simulink model "Balancing Model"  (R2024a)
settings: Solver=VariableStepAuto  StartTime=0.0  StopTime=inf  RelTol=1e-3
settings Model: Creator=Ganna Ayman  LastModifiedBy=Ganna Ayman

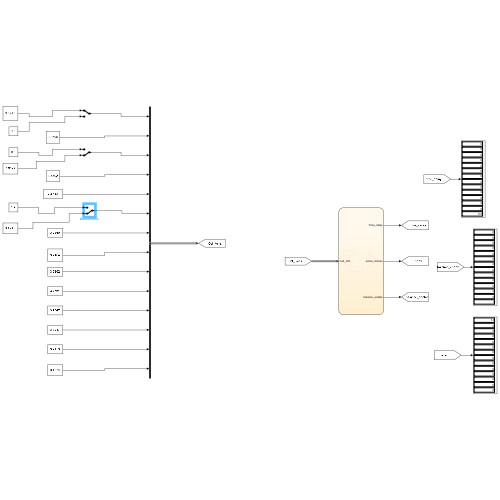
[thumbnail: Simulink's stored preview of the top-level diagram]
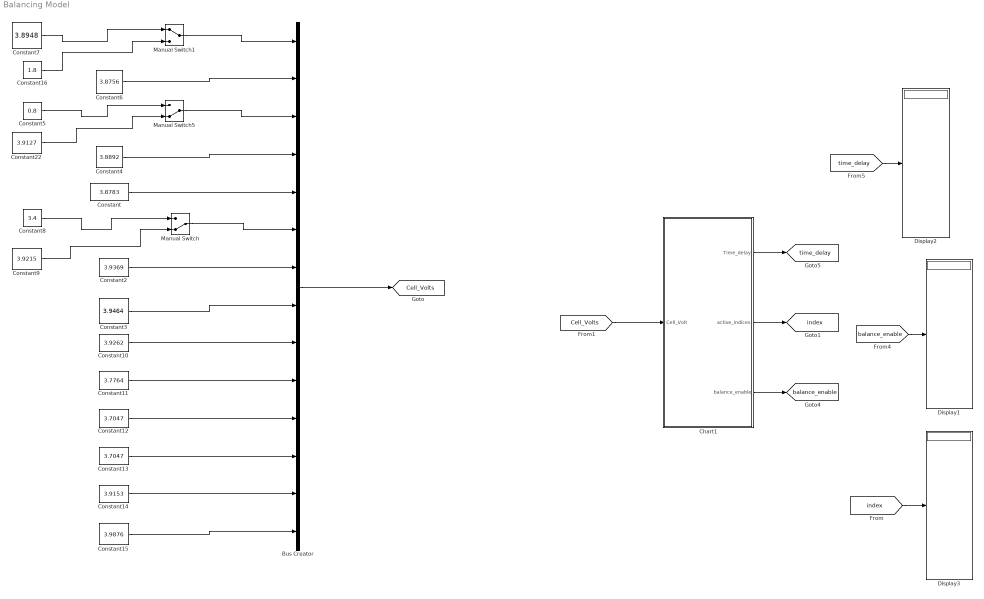
== system Balancing Model ==
  Bus Creator : BusCreator  Inputs=14
  Chart1 : Stateflow chart  TreatAsAtomicUnit=on
      settings: PortSchema="{\"entries\":[{\"content\":{\"sides\":[{\"content\":{\"connectorIds\":[\"In1\"]},\"type\":\"ConnectorPlacement.EquallySpacedRectSide\",\"uuid\":\"6f312cc7-79af-4024-8579-3732173f9295\"},{\"content\":{\"connectorIds\":[\"Out2\",\"Out3\",\"Out1\"],\"side\":\"RIGHT\"},\"type\":\"ConnectorPlacement.EquallySpacedRectSide\",\"uuid\":\"3dc9c74e-fd1a-461c-96fc-bb153941e7b5\"},{\"content\":{\"side\":\"TOP\"},\"type\":\"ConnectorPlacement.EquallySpacedRectSide\",\"uuid\":\"e4504d25-18f4-45f4-b711-d682a6c51dcf\"}]},\"type\":\"ConnectorPlacement.EquallySpacedConnector\",\"uuid\":\"9caf59e1-89f7-43be-b634-7a97cd583662\"}],\"packageUris\":[\"http://schema.mathworks.com/mf0/Connector/R2020b\"],\"version\":\"1.0\"}"
  Constant : Constant  Value=3.8783
  Constant10 : Constant  Value=3.9262
  Constant11 : Constant  Value=3.7764
  Constant12 : Constant  Value=3.7047
  Constant13 : Constant  Value=3.7047
  Constant14 : Constant  Value=3.9153
  Constant15 : Constant  Value=3.9876
  Constant16 : Constant  Value=1.8
  Constant2 : Constant  Value=3.9369
  Constant22 : Constant  Value=3.9127
  Constant3 : Constant  Value=3.9464
  Constant4 : Constant  Value=3.8892
  Constant5 : Constant  Value=0.8
  Constant6 : Constant  Value=3.8756
  Constant7 : Constant  Value=3.8948
  Constant8 : Constant  Value=3.4
  Constant9 : Constant  Value=3.9215
  Display1 : Display
  Display2 : Display
  Display3 : Display
  Manual Switch : ManualSwitch  CurrentSetting=0
  Manual Switch1 : ManualSwitch
  Manual Switch5 : ManualSwitch  CurrentSetting=0
  tag scope: Cell_Volts=global, balance_enable=global, index=global, time_delay=global
  wires:
  Constant8/1 -> Manual Switch/1
  [balance_enable] -> Display1/1
  Constant10/1 -> Bus Creator/9
  Constant5/1 -> Manual Switch5/1
  [time_delay] -> Display2/1
  Constant4/1 -> Bus Creator/4
  Chart1/1(balance_enable) -> [balance_enable]
  Constant2/1 -> Bus Creator/7
  Manual Switch/1 -> Bus Creator/6
  Constant16/1 -> Manual Switch1/2
  Constant/1 -> Bus Creator/5
  Constant12/1 -> Bus Creator/11
  Bus Creator/1 -> [Cell_Volts]
  Constant3/1 -> Bus Creator/8
  Constant6/1 -> Bus Creator/2
  Constant11/1 -> Bus Creator/10
  Constant13/1 -> Bus Creator/12
  Constant7/1 -> Manual Switch1/1
  Constant15/1 -> Bus Creator/14
  Constant9/1 -> Manual Switch/2
  Constant14/1 -> Bus Creator/13
  Constant22/1 -> Manual Switch5/2
  Manual Switch5/1 -> Bus Creator/3
  Manual Switch1/1 -> Bus Creator/1
  Chart1/2(Time_delay) -> [time_delay]
  [index] -> Display3/1
  Chart1/3(active_indices) -> [index]
  [Cell_Volts] -> Chart1/1(Cell_Volt)

== stateflow chart Balancing Model/Chart1 ==
  state Discharge_Time_interval
    H= 1;
    Time_delay = zeros(1, 14);  % Initialize array
    during:
    for H = 1:14
    if balance_enable(H) == 1
    Time_delay(H) = 0.5; % 0.5min
    else
    Time_delay(H) = 0;      % 0 if disabled
    end
    end
    exit:
    H=1;
  state initialization
    entry:
    balance_enable=zeros(1,14);
    n=1;
    i=1;
    G=1;
    H=1;
  state Get_balance_reference
    entry:
    i=1
    cell_reference=10;
    during :
    for i = 1:14
    if (Cell_Volt(i) < cell_reference) && (Cell_Volt(i)>1.5)
    cell_reference = Cell_Volt(i);
    end
    end;
    exit:
    i=1;
  state Index_number
    entry:
    active_indices = zeros(1,14);  % Initialize output
    idx = 1;                     % Counter for active indices
    during:
    for G = 1:14
    if balance_enable(G) == 1
    active_indices(idx) = G;  % Store cell
    idx = idx + 1;
    end
    end
    exit:
    G=1;
  state Data_Check
    i = 1;
    % Main loop
    for i = 1:14
    if (Cell_Volt(i) > cell_reference) && (Cell_Volt(i) > 1.6) &&(Cell_Volt(i) - cell_reference > 0.25)
    balance_enable(i) = 1;
    else
    balance_enable(i) = 0; %had5ol feha 3and as8ar wa7da + lo el difference kan akber mn 0.25
    end
    end
    exit :
    i=1;
  state Error_Check
    entry:
    abdullah = 0;  % Initialize output (0 by default)
    during:
    for G = 1:14
    % Calculate absolute difference
    diff = abs(Cell_Volt(G) - cell_reference);
    % Check condition
    if diff > 0.5
    abdullah = 1;  % Set flag
    end
    end
    end
    exit:
    G=1;
  (default) -> initialization
  Discharge_Time_interval -> Get_balance_reference : after(30,sec)[(H==14)]
  initialization -> Get_balance_reference
  Index_number -> Discharge_Time_interval : [G==14]
  Error_Check -> Get_balance_reference [order 2] : [abdullah==1]
  Get_balance_reference -> Error_Check : [i==14]
  Data_Check -> Index_number : [i==14]
  Error_Check -> Data_Check [order 1] : [(G==14)&&(abdullah==0)]
  data: Cell_Volt input double size=[1,14]; balance_enable output double size=[1,14]; i local; G local; H local; n local; cell_reference local; Time_delay output double size=[1,14]; active_indices output double size=[1,14]; idx local; abdullah local; diff local
